simulink model "tailsitter2019b"  (R2019b)
settings: Solver=VariableStepAuto  StartTime=0.0  StopTime=10  RelTol=1e-3
values from neighbouring files (symbols this model uses):
  A_R = b^2/S    (= 3.125)    [tailsitterParam.m]
  b = [b1;b2;b3;b4;b5;b4;b3]    [tailsitterParam.m]
  c = [c1;c2;c3;c3;c3;c3;c3]    [tailsitterParam.m]
  C_D0 = 0.02    [tailsitterParam.m]
  C_D_R = 1.1    [tailsitterParam.m]
  C_M_coeff = polyfit(C_M_alpha(:,1), C_M_alpha(:,2),3)    [tailsitterParam.m]
  Cl_alpha = (2*pi*cos(Lambda))/(2*cos(Lambda)/A_R + sqrt(1 + (2*cos(Lambda)/A_R)^2))    [tailsitterParam.m]
  d = cat(2,p_d,p_d)    [tailsitterParam.m]
  g = -9.82    [tailsitterParam.m]
  Ic = [Ix 0 -Ixz;0 Iy 0;-Ixz 0 Iz]    [tailsitterParam.m]
  Initial_coeffs = polyfit(Thrusts_0,Omegas_0,4)    [tailsitterParam.m]
  Ith = 1.6*10^(-6)    (= 1.6e-06)    [tailsitterParam.m]
  k0 = 0.87    [tailsitterParam.m]
  l = 0.145    [tailsitterParam.m]
  li = cat(2,lr,ll)    [tailsitterParam.m]
  m = 0.21    [tailsitterParam.m]
  M_inv = inv(M)    [tailsitterParam.m]
  Omega_max = 1500    [tailsitterParam.m]
  pm = cat(2,prm,plm)    [tailsitterParam.m]
  r_B = r_B./1000    [tailsitterParam.m]
  R_eb = axang2rotm([0 1 0 -1.572])    [tailsitterParam.m]
  R_eleb1 = axang2rotm([0 0 1 -0.16349])    [tailsitterParam.m]
  R_eleb2 = axang2rotm([0 0 1 0.15331])    [tailsitterParam.m]
  rho = 1.225    [tailsitterParam.m]
  rp = 0.0625    [tailsitterParam.m]
  rv_B = rv_B./1000    [tailsitterParam.m]
  t_be = [0.5;0;0.5]    [tailsitterParam.m]
libraries: simulink x6, vrlib x1
settings Model: Creator=Thobi  LastModifiedBy=morten
settings DebuggingCC: SFMachineParentedDataDiag=error

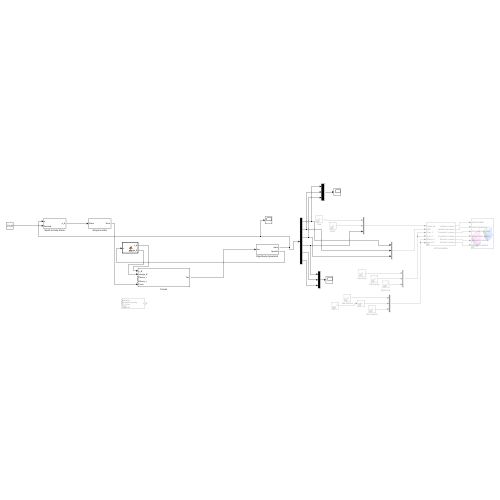
[thumbnail: Simulink's stored preview of the top-level diagram]
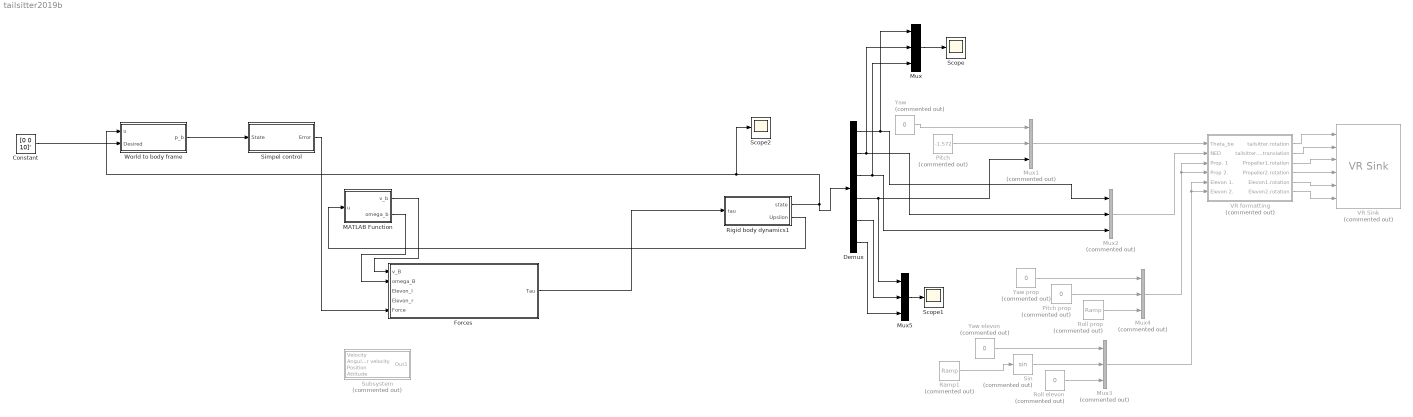
== system tailsitter2019b ==
  Constant : Constant  Value=[0 0 10]'
  Demux : Demux  Outputs=6
  Forces : Subsystem
  MATLAB Function : MATLAB Function  TreatAsAtomicUnit=on
  Mux : Mux  Inputs=3
  Mux{1..4} (4 alike) : Mux  Commented=on  Inputs=3
  Mux5 : Mux  Inputs=3
  Pitch : Constant  Commented=on  Value=-1.572
  Pitch prop : Constant  Commented=on  Value=0
  Ramp1 : simulink/Sources/Ramp  Commented=on  slope=1  start=0  InitialOutput=0
  Rigid body dynamics1 : Subsystem
  Roll elevon : Constant  Commented=on  Value=0
  Roll prop : simulink/Sources/Ramp  Commented=on  slope=1  start=0  InitialOutput=0
  Scope : Scope
  Scope1 : Scope
  Scope2 : Scope
  Simpel control : Subsystem
  Sin : Trigonometry  Commented=on
  Subsystem : Subsystem  Commented=on
  VR Sink : vrlib/VR Sink  Commented=on  InstantiateOnLoad=on  SampleTime=0.1  ViewEnable=on  RemoteChange=off  RemoteView=on  FieldsWritten=UAV.rotation.4.1.1.double#UAV.translation.3.1.1.double#Propeller1.rotation.4.1.1.double#Propeller2.rotation.4.1.1.double#Elevon1.rotation.4.1.1.double#Elevon2.rotation.4.1.1.double  WorldFileName=tailsitter_VR_simple.x3d  AutoView=off  VideoDimensions=[]  AllowVariableSize=off
  VR formatting : Subsystem  Commented=on
  World to body frame : Subsystem
  Yaw : Constant  Commented=on  Value=0
  Yaw elevon : Constant  Commented=on  Value=0
  Yaw prop : Constant  Commented=on  Value=0
  wires:
  VR formatting/5(Elevon1.rotation) -> VR Sink/5
  Roll prop/1 -> Mux4/3
  VR formatting/1(tailsitter.rotation) -> VR Sink/1
  Mux1/1 -> VR formatting/1(Theta_be)
  VR formatting/2(tailsitter.translation) -> VR Sink/2
  Sin/1 -> Mux3/2
  Roll elevon/1 -> Mux3/3
  Ramp1/1 -> Sin/1
  Yaw elevon/1 -> Mux3/1
  Mux3/1 -> VR formatting/6(Elevon 2.), VR formatting/5(Elevon 1.)
  Rigid body dynamics1/1(state) -> Demux/1, Scope2/1, World to body frame/1(u)
  Pitch/1 -> Mux1/2
  Demux/2 -> Mux/2, Mux2/2
  Mux2/1 -> VR formatting/2(NED)
  Yaw/1 -> Mux1/1
  VR formatting/6(Elevon2.rotation) -> VR Sink/6
  VR formatting/4(Propeller2.rotation) -> VR Sink/4
  Demux/4 -> Mux5/1, Mux1/3
  Yaw prop/1 -> Mux4/1
  Pitch prop/1 -> Mux4/2
  VR formatting/3(Propeller1.rotation) -> VR Sink/3
  Mux4/1 -> VR formatting/4(Prop 2.), VR formatting/3("Prop. 1 ")
  Simpel control/1(Error) -> Forces/5(Force)
  World to body frame/1(p_b) -> Simpel control/1(State)
  Rigid body dynamics1/2(Upsilon) -> MATLAB Function/1(u)
  MATLAB Function/1(v_b) -> Forces/1(v_B)
  MATLAB Function/2(omega_b) -> Forces/2(omega_B)
  Forces/1(Tau) -> Rigid body dynamics1/1(tau)
  Demux/1 -> Mux/1, Mux2/1
  Demux/3 -> Mux/3, Mux2/3
  Mux/1 -> Scope/1
  Demux/5 -> Mux5/2
  Demux/6 -> Mux5/3
  Mux5/1 -> Scope1/1
  Constant/1 -> World to body frame/2(Desired)

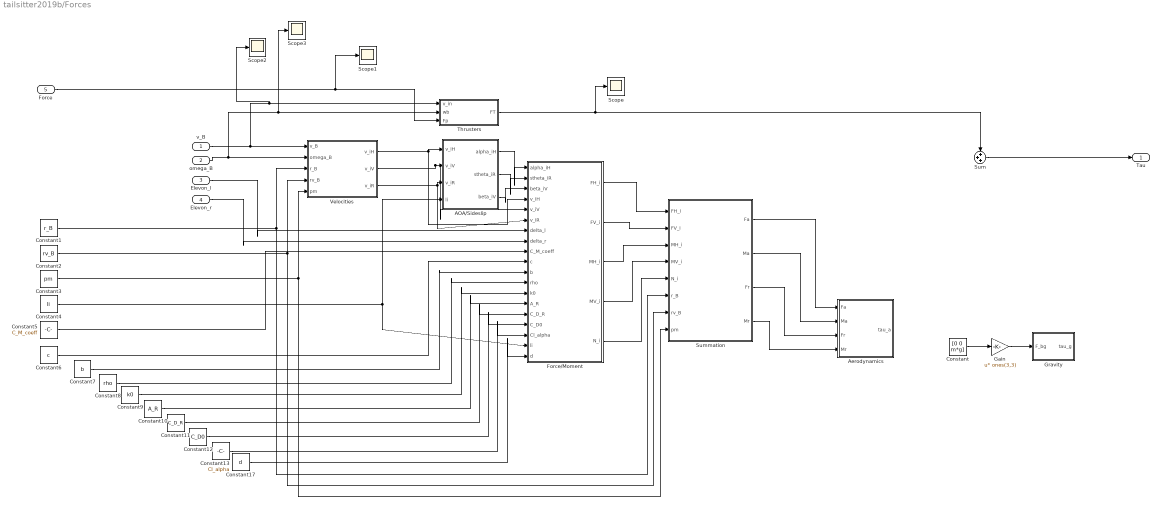
== system tailsitter2019b/Forces ==
  v_B : Inport
  omega_B : Inport  Port=2
  Elevon_l : Inport  Port=3
  Elevon_r : Inport  Port=4
  Force : Inport  Port=5
  AOA/Sideslip : MATLAB Function  TreatAsAtomicUnit=on
  Aerodynamics : MATLAB Function  TreatAsAtomicUnit=on
  Constant : Constant  Value=[0 0 m*g]
  Constant1 : Constant  Value=r_B
  Constant10 : Constant  Value=A_R
  Constant11 : Constant  Value=C_D_R
  Constant12 : Constant  Value=C_D0
  Constant13 : Constant  Value=Cl_alpha
  Constant17 : Constant  Value=d
  Constant2 : Constant  Value=rv_B
  Constant3 : Constant  Value=pm
  Constant4 : Constant  Value=li
  Constant5 : Constant  Value=C_M_coeff
  Constant6 : Constant  Value=c
  Constant7 : Constant  Value=b
  Constant8 : Constant  Value=rho
  Constant9 : Constant  Value=k0
  Force/Moment : MATLAB Function  TreatAsAtomicUnit=on
  Gain : Gain  Gain=ones(3,3)  Multiplication=Matrix(u*K)
  Gravity : MATLAB Function  TreatAsAtomicUnit=on
  Scope{,1..3} (4 alike) : Scope
  Sum : Sum  Inputs=+++
  Summation : MATLAB Function  TreatAsAtomicUnit=on
  Thrusters : Subsystem
  Velocities : MATLAB Function  TreatAsAtomicUnit=on
  Tau : Outport
  wires:
  v_B/1 -> Scope2/1, Thrusters/1(v_in), Velocities/1(v_B)
  Gain/1 -> Gravity/1(F_bg)
  Velocities/1(v_iH) -> AOA/Sideslip/1(v_iH), Force/Moment/4(v_iH)
  Velocities/2(v_iV) -> Force/Moment/5(v_iV), AOA/Sideslip/2(v_iV)
  Velocities/3(v_iR) -> Force/Moment/6(v_iR), AOA/Sideslip/3(v_iR)
  AOA/Sideslip/1(alpha_iH) -> Force/Moment/1(alpha_iH)
  AOA/Sideslip/2(stheta_iR) -> Force/Moment/2(stheta_iR)
  AOA/Sideslip/3(beta_iV) -> Force/Moment/3(beta_iV)
  Force/Moment/1(FH_i) -> Summation/1(FH_i)
  Force/Moment/2(FV_i) -> Summation/2(FV_i)
  Force/Moment/3(MH_i) -> Summation/3(MH_i)
  Force/Moment/4(MV_i) -> Summation/4(MV_i)
  Force/Moment/5(N_i) -> Summation/5(N_i)
  Summation/1(Fa) -> Aerodynamics/1(Fa)
  Summation/2(Ma) -> Aerodynamics/2(Ma)
  Summation/3(Fr) -> Aerodynamics/3(Fr)
  Summation/4(Mr) -> Aerodynamics/4(Mr)
  Sum/1 -> Tau/1
  Elevon_l/1 -> Force/Moment/7(delta_l)
  Elevon_r/1 -> Force/Moment/8(delta_r)
  Constant/1 -> Gain/1
  Constant1/1 -> Summation/6(r_B), Velocities/3(r_B)
  Constant2/1 -> Velocities/4(rv_B), Summation/7(rv_B)
  Constant3/1 -> Velocities/5(pm), Summation/8(pm)
  Constant4/1 -> Force/Moment/18(li), AOA/Sideslip/4(li)
  Constant5/1 -> Force/Moment/9(C_M_coeff)
  Constant6/1 -> Force/Moment/10(c)
  Constant7/1 -> Force/Moment/11(b)
  Constant8/1 -> Force/Moment/12(rho)
  Constant9/1 -> Force/Moment/13(k0)
  Constant10/1 -> Force/Moment/14(A_R)
  Constant11/1 -> Force/Moment/15(C_D_R)
  Constant12/1 -> Force/Moment/16(C_D0)
  Constant13/1 -> Force/Moment/17(Cl_alpha)
  Thrusters/1(FT) -> Scope/1, Sum/1
  Constant17/1 -> Force/Moment/19(d)
  Force/1 -> Scope1/1, Thrusters/3(Fp)
  omega_B/1 -> Thrusters/2(wb), Scope3/1, Velocities/2(omega_B)

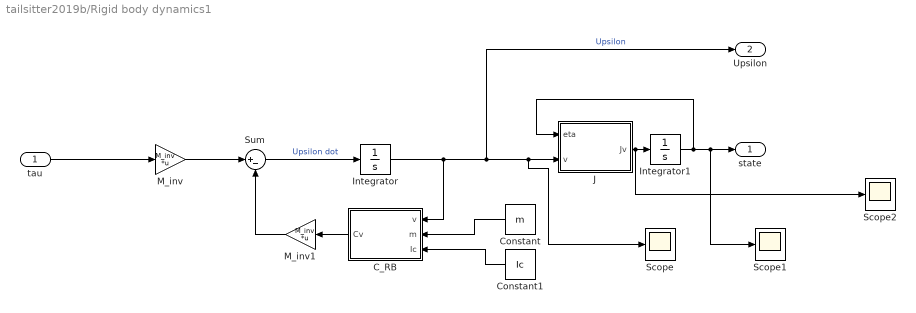
== system tailsitter2019b/Rigid body dynamics1 ==
  tau : Inport
  C_RB : MATLAB Function  TreatAsAtomicUnit=on
  Constant : Constant  Value=m
  Constant1 : Constant  Value=Ic
  Integrator : Integrator  InitialCondition=[0;0;0;0;0;0]
  Integrator1 : Integrator  InitialCondition=[0;0;0;0;-pi/2;0]
  J : MATLAB Function  TreatAsAtomicUnit=on
  M_inv : Gain  Gain=M_inv  Multiplication=Matrix(K*u) (u vector)
  M_inv1 : Gain  Gain=M_inv  Multiplication=Matrix(K*u) (u vector)
  Scope : Scope
  Scope1 : Scope
  Scope2 : Scope
  Sum : Sum  Inputs=|+-
  state : Outport
  Upsilon : Outport  Port=2
  wires:
  tau/1 -> M_inv/1
  M_inv/1 -> Sum/1
  Sum/1 -> Integrator/1  "Upsilon dot"
  C_RB/1(Cv) -> M_inv1/1
  M_inv1/1 -> Sum/2
  Integrator/1 -> C_RB/1(v), Upsilon/1, Scope/1, J/2(v)  "Upsilon"
  Constant/1 -> C_RB/2(m)
  Constant1/1 -> C_RB/3(Ic)
  J/1(Jv) -> Scope2/1, Integrator1/1
  Integrator1/1 -> Scope1/1, state/1, J/1(eta)

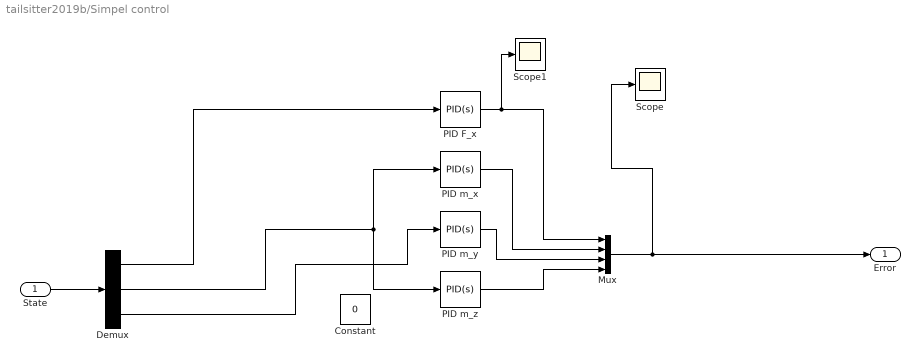
== system tailsitter2019b/Simpel control ==
  State : Inport
  Constant : Constant  Value=0
  Demux : Demux  Outputs=3
  Mux : Mux
  PID F_x : simulink/Continuous/PID Controller  Controller=PID  Form=Parallel  TimeDomain=Continuous-time  SampleTime=-1  IntegratorMethod=Forward Euler  ControllerParametersSource=internal  P=1.2  I=1  D=0  UseFilter=on  N=100  TunerSelectOption=Transfer Function Based (PID Tuner App)  InitialConditionSource=internal  InitialConditionForIntegrator=0  InitialConditionForFilter=0  DifferentiatorICPrevScaledInput=0  ExternalReset=none  TrackingMode=off  Kt=1  LimitOutput=off  UpperSaturationLimit=inf  LowerSaturationLimit=-inf  LinearizeAsGain=on  AntiWindupMode=none  Kb=1  POutMin=[]  POutMax=[]  IOutMin=[]  IOutMax=[]  DOutMin=[]  DOutMax=[]  NOutMin=[]  NOutMax=[]  SumOutMin=[]  SumOutMax=[]  SaturationOutMin=[]  SaturationOutMax=[]  PParamMin=[]  PParamMax=[]  IParamMin=[]  IParamMax=[]  DParamMin=[]  DParamMax=[]  NParamMin=[]  NParamMax=[]  KbParamMin=[]  KbParamMax=[]  KtParamMin=[]  KtParamMax=[]  KbOutMin=[]  KbOutMax=[]  KtOutMin=[]  KtOutMax=[]  IntegratorOutMin=[]  IntegratorOutMax=[]  FilterOutMin=[]  FilterOutMax=[]  SumI1OutMin=[]  SumI1OutMax=[]  SumI2OutMin=[]  SumI2OutMax=[]  SumI3OutMin=[]  SumI3OutMax=[]  SumI4OutMin=[]  SumI4OutMax=[]  SumDOutMin=[]  SumDOutMax=[]  DifferentiatorOutMin=[]  DifferentiatorOutMax=[]  FilterDiffOutCoefMin=[]  FilterDiffOutCoefMax=[]  ReciprocalOutMin=[]  ReciprocalOutMax=[]  SumDenOutMin=[]  SumDenOutMax=[]  SumNumOutMin=[]  SumNumOutMax=[]  DivideOutMin=[]  DivideOutMax=[]  IntegratorContinuousStateAttributes=''  IntegratorStateMustResolveToSignalObject=off  IntegratorRTWStateStorageClass=Auto  FilterContinuousStateAttributes=''  FilterStateMustResolveToSignalObject=off  FilterRTWStateStorageClass=Auto  ParallelPVariant=InternalParameters  IdealPVariant=Disabled  IVariant=InternalParameters  DVariant=InternalParameters  IntegratorVariant=Continuous  SatVariant=Disabled  AWVariant=Passthrough  PCopyVariant=Disabled  TRVariant=Disabled  FdbkBlocksVariant=Forward  IdealPFdbkVariant=Disabled  SatFdbkVariant=Disabled  DerivativeFilterVariant=ContFilter  NVariant=InternalParameters  NCopyVariant=Disabled  FilterICVariant=InternalICsFilter  IntegratorICVariant=InternalICs  ExternalResetVariant=Disabled  TRSumVariant=Passthrough  SumFdbkVariant=Disabled  SumVariant=Sum_PID
  PID m_x : simulink/Continuous/PID Controller  Controller=PID  Form=Parallel  TimeDomain=Continuous-time  SampleTime=-1  IntegratorMethod=Forward Euler  ControllerParametersSource=internal  P=1.2  I=1  D=0  UseFilter=on  N=100  TunerSelectOption=Transfer Function Based (PID Tuner App)  InitialConditionSource=internal  InitialConditionForIntegrator=0  InitialConditionForFilter=0  DifferentiatorICPrevScaledInput=0  ExternalReset=none  TrackingMode=off  Kt=1  LimitOutput=off  UpperSaturationLimit=inf  LowerSaturationLimit=-inf  LinearizeAsGain=on  AntiWindupMode=none  Kb=1  POutMin=[]  POutMax=[]  IOutMin=[]  IOutMax=[]  DOutMin=[]  DOutMax=[]  NOutMin=[]  NOutMax=[]  SumOutMin=[]  SumOutMax=[]  SaturationOutMin=[]  SaturationOutMax=[]  PParamMin=[]  PParamMax=[]  IParamMin=[]  IParamMax=[]  DParamMin=[]  DParamMax=[]  NParamMin=[]  NParamMax=[]  KbParamMin=[]  KbParamMax=[]  KtParamMin=[]  KtParamMax=[]  KbOutMin=[]  KbOutMax=[]  KtOutMin=[]  KtOutMax=[]  IntegratorOutMin=[]  IntegratorOutMax=[]  FilterOutMin=[]  FilterOutMax=[]  SumI1OutMin=[]  SumI1OutMax=[]  SumI2OutMin=[]  SumI2OutMax=[]  SumI3OutMin=[]  SumI3OutMax=[]  SumI4OutMin=[]  SumI4OutMax=[]  SumDOutMin=[]  SumDOutMax=[]  DifferentiatorOutMin=[]  DifferentiatorOutMax=[]  FilterDiffOutCoefMin=[]  FilterDiffOutCoefMax=[]  ReciprocalOutMin=[]  ReciprocalOutMax=[]  SumDenOutMin=[]  SumDenOutMax=[]  SumNumOutMin=[]  SumNumOutMax=[]  DivideOutMin=[]  DivideOutMax=[]  IntegratorContinuousStateAttributes=''  IntegratorStateMustResolveToSignalObject=off  IntegratorRTWStateStorageClass=Auto  FilterContinuousStateAttributes=''  FilterStateMustResolveToSignalObject=off  FilterRTWStateStorageClass=Auto  ParallelPVariant=InternalParameters  IdealPVariant=Disabled  IVariant=InternalParameters  DVariant=InternalParameters  IntegratorVariant=Continuous  SatVariant=Disabled  AWVariant=Passthrough  PCopyVariant=Disabled  TRVariant=Disabled  FdbkBlocksVariant=Forward  IdealPFdbkVariant=Disabled  SatFdbkVariant=Disabled  DerivativeFilterVariant=ContFilter  NVariant=InternalParameters  NCopyVariant=Disabled  FilterICVariant=InternalICsFilter  IntegratorICVariant=InternalICs  ExternalResetVariant=Disabled  TRSumVariant=Passthrough  SumFdbkVariant=Disabled  SumVariant=Sum_PID
  PID m_y : simulink/Continuous/PID Controller  Controller=PID  Form=Parallel  TimeDomain=Continuous-time  SampleTime=-1  IntegratorMethod=Forward Euler  ControllerParametersSource=internal  P=1.2  I=1  D=0  UseFilter=on  N=100  TunerSelectOption=Transfer Function Based (PID Tuner App)  InitialConditionSource=internal  InitialConditionForIntegrator=0  InitialConditionForFilter=0  DifferentiatorICPrevScaledInput=0  ExternalReset=none  TrackingMode=off  Kt=1  LimitOutput=off  UpperSaturationLimit=inf  LowerSaturationLimit=-inf  LinearizeAsGain=on  AntiWindupMode=none  Kb=1  POutMin=[]  POutMax=[]  IOutMin=[]  IOutMax=[]  DOutMin=[]  DOutMax=[]  NOutMin=[]  NOutMax=[]  SumOutMin=[]  SumOutMax=[]  SaturationOutMin=[]  SaturationOutMax=[]  PParamMin=[]  PParamMax=[]  IParamMin=[]  IParamMax=[]  DParamMin=[]  DParamMax=[]  NParamMin=[]  NParamMax=[]  KbParamMin=[]  KbParamMax=[]  KtParamMin=[]  KtParamMax=[]  KbOutMin=[]  KbOutMax=[]  KtOutMin=[]  KtOutMax=[]  IntegratorOutMin=[]  IntegratorOutMax=[]  FilterOutMin=[]  FilterOutMax=[]  SumI1OutMin=[]  SumI1OutMax=[]  SumI2OutMin=[]  SumI2OutMax=[]  SumI3OutMin=[]  SumI3OutMax=[]  SumI4OutMin=[]  SumI4OutMax=[]  SumDOutMin=[]  SumDOutMax=[]  DifferentiatorOutMin=[]  DifferentiatorOutMax=[]  FilterDiffOutCoefMin=[]  FilterDiffOutCoefMax=[]  ReciprocalOutMin=[]  ReciprocalOutMax=[]  SumDenOutMin=[]  SumDenOutMax=[]  SumNumOutMin=[]  SumNumOutMax=[]  DivideOutMin=[]  DivideOutMax=[]  IntegratorContinuousStateAttributes=''  IntegratorStateMustResolveToSignalObject=off  IntegratorRTWStateStorageClass=Auto  FilterContinuousStateAttributes=''  FilterStateMustResolveToSignalObject=off  FilterRTWStateStorageClass=Auto  ParallelPVariant=InternalParameters  IdealPVariant=Disabled  IVariant=InternalParameters  DVariant=InternalParameters  IntegratorVariant=Continuous  SatVariant=Disabled  AWVariant=Passthrough  PCopyVariant=Disabled  TRVariant=Disabled  FdbkBlocksVariant=Forward  IdealPFdbkVariant=Disabled  SatFdbkVariant=Disabled  DerivativeFilterVariant=ContFilter  NVariant=InternalParameters  NCopyVariant=Disabled  FilterICVariant=InternalICsFilter  IntegratorICVariant=InternalICs  ExternalResetVariant=Disabled  TRSumVariant=Passthrough  SumFdbkVariant=Disabled  SumVariant=Sum_PID
  PID m_z : simulink/Continuous/PID Controller  Controller=PID  Form=Parallel  TimeDomain=Continuous-time  SampleTime=-1  IntegratorMethod=Forward Euler  ControllerParametersSource=internal  P=1.2  I=1  D=0  UseFilter=on  N=100  TunerSelectOption=Transfer Function Based (PID Tuner App)  InitialConditionSource=internal  InitialConditionForIntegrator=0  InitialConditionForFilter=0  DifferentiatorICPrevScaledInput=0  ExternalReset=none  TrackingMode=off  Kt=1  LimitOutput=off  UpperSaturationLimit=inf  LowerSaturationLimit=-inf  LinearizeAsGain=on  AntiWindupMode=none  Kb=1  POutMin=[]  POutMax=[]  IOutMin=[]  IOutMax=[]  DOutMin=[]  DOutMax=[]  NOutMin=[]  NOutMax=[]  SumOutMin=[]  SumOutMax=[]  SaturationOutMin=[]  SaturationOutMax=[]  PParamMin=[]  PParamMax=[]  IParamMin=[]  IParamMax=[]  DParamMin=[]  DParamMax=[]  NParamMin=[]  NParamMax=[]  KbParamMin=[]  KbParamMax=[]  KtParamMin=[]  KtParamMax=[]  KbOutMin=[]  KbOutMax=[]  KtOutMin=[]  KtOutMax=[]  IntegratorOutMin=[]  IntegratorOutMax=[]  FilterOutMin=[]  FilterOutMax=[]  SumI1OutMin=[]  SumI1OutMax=[]  SumI2OutMin=[]  SumI2OutMax=[]  SumI3OutMin=[]  SumI3OutMax=[]  SumI4OutMin=[]  SumI4OutMax=[]  SumDOutMin=[]  SumDOutMax=[]  DifferentiatorOutMin=[]  DifferentiatorOutMax=[]  FilterDiffOutCoefMin=[]  FilterDiffOutCoefMax=[]  ReciprocalOutMin=[]  ReciprocalOutMax=[]  SumDenOutMin=[]  SumDenOutMax=[]  SumNumOutMin=[]  SumNumOutMax=[]  DivideOutMin=[]  DivideOutMax=[]  IntegratorContinuousStateAttributes=''  IntegratorStateMustResolveToSignalObject=off  IntegratorRTWStateStorageClass=Auto  FilterContinuousStateAttributes=''  FilterStateMustResolveToSignalObject=off  FilterRTWStateStorageClass=Auto  ParallelPVariant=InternalParameters  IdealPVariant=Disabled  IVariant=InternalParameters  DVariant=InternalParameters  IntegratorVariant=Continuous  SatVariant=Disabled  AWVariant=Passthrough  PCopyVariant=Disabled  TRVariant=Disabled  FdbkBlocksVariant=Forward  IdealPFdbkVariant=Disabled  SatFdbkVariant=Disabled  DerivativeFilterVariant=ContFilter  NVariant=InternalParameters  NCopyVariant=Disabled  FilterICVariant=InternalICsFilter  IntegratorICVariant=InternalICs  ExternalResetVariant=Disabled  TRSumVariant=Passthrough  SumFdbkVariant=Disabled  SumVariant=Sum_PID
  Scope : Scope
  Scope1 : Scope
  Error : Outport
  wires:
  Mux/1 -> Scope/1, Error/1
  Demux/1 -> PID F_x/1
  State/1 -> Demux/1
  Demux/2 -> PID m_z/1, PID m_x/1
  Demux/3 -> PID m_y/1
  PID F_x/1 -> Scope1/1, Mux/1
  PID m_x/1 -> Mux/2
  PID m_y/1 -> Mux/3
  PID m_z/1 -> Mux/4

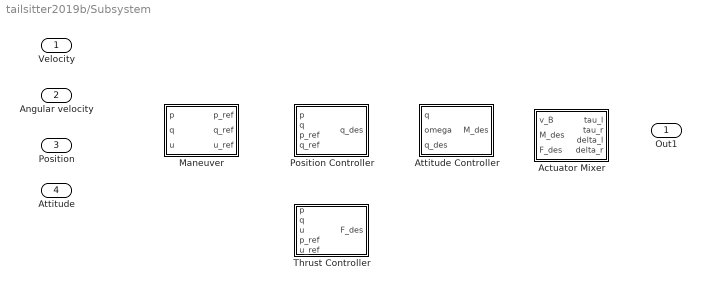
== system tailsitter2019b/Subsystem ==
  Velocity : Inport
  Angular velocity : Inport  Port=2
  Position : Inport  Port=3
  Attitude : Inport  Port=4
  Actuator Mixer : MATLAB Function  TreatAsAtomicUnit=on
  Attitude Controller : MATLAB Function  TreatAsAtomicUnit=on
  Maneuver : MATLAB Function  TreatAsAtomicUnit=on
  Position Controller : MATLAB Function  TreatAsAtomicUnit=on
  Thrust Controller : MATLAB Function  TreatAsAtomicUnit=on
  Out1 : Outport

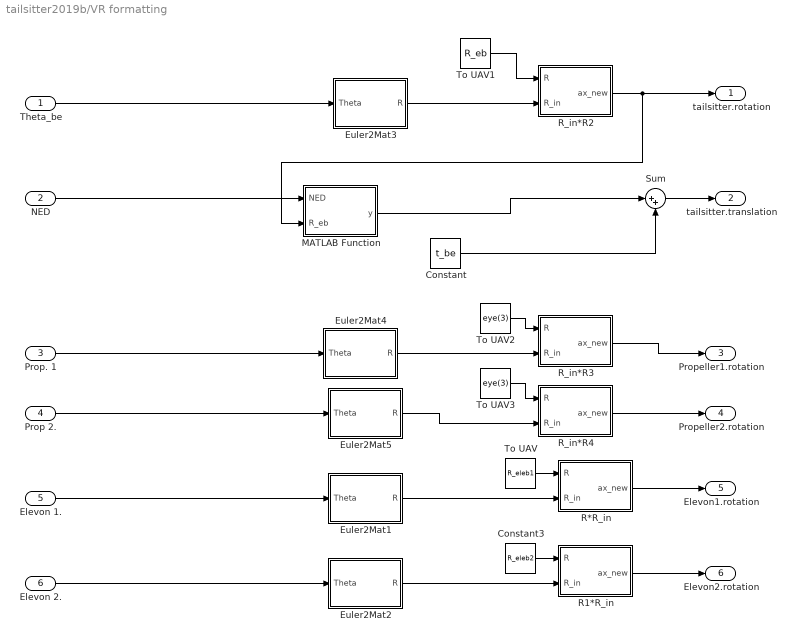
== system tailsitter2019b/VR formatting ==
  Theta_be : Inport
  NED : Inport  Port=2
  "Prop. 1 " : Inport  Port=3
  Prop 2. : Inport  Port=4
  Elevon 1. : Inport  Port=5
  Elevon 2. : Inport  Port=6
  Constant : Constant  Value=t_be
  Constant3 : Constant  Value=R_eleb2
  Euler2Mat1 : MATLAB Function  TreatAsAtomicUnit=on
  Euler2Mat2 : MATLAB Function  TreatAsAtomicUnit=on
  Euler2Mat3 : MATLAB Function  TreatAsAtomicUnit=on
  Euler2Mat4 : MATLAB Function  TreatAsAtomicUnit=on
  Euler2Mat5 : MATLAB Function  TreatAsAtomicUnit=on
  MATLAB Function : MATLAB Function  TreatAsAtomicUnit=on
  R*R_in : MATLAB Function  TreatAsAtomicUnit=on
  R1*R_in : MATLAB Function  TreatAsAtomicUnit=on
  R_in*R2 : MATLAB Function  TreatAsAtomicUnit=on
  R_in*R3 : MATLAB Function  TreatAsAtomicUnit=on
  R_in*R4 : MATLAB Function  TreatAsAtomicUnit=on
  Sum : Sum  Inputs=|++
  To UAV : Constant  Value=R_eleb1
  To UAV1 : Constant  Value=R_eb
  To UAV2 : Constant  Value=eye(3)
  To UAV3 : Constant  Value=eye(3)
  tailsitter.rotation : Outport
  tailsitter.translation : Outport  Port=2
  Propeller1.rotation : Outport  Port=3
  Propeller2.rotation : Outport  Port=4
  Elevon1.rotation : Outport  Port=5
  Elevon2.rotation : Outport  Port=6
  wires:
  NED/1 -> MATLAB Function/1(NED)
  Theta_be/1 -> Euler2Mat3/1(Theta)
  MATLAB Function/1(y) -> Sum/1
  Sum/1 -> tailsitter.translation/1
  Constant/1 -> Sum/2
  "Prop. 1 "/1 -> Euler2Mat4/1(Theta)
  Elevon 1./1 -> Euler2Mat1/1(Theta)
  Elevon 2./1 -> Euler2Mat2/1(Theta)
  Euler2Mat1/1(R) -> R*R_in/2(R_in)
  To UAV/1 -> R*R_in/1(R)
  R*R_in/1(ax_new) -> Elevon1.rotation/1
  Euler2Mat2/1(R) -> R1*R_in/2(R_in)
  R1*R_in/1(ax_new) -> Elevon2.rotation/1
  Constant3/1 -> R1*R_in/1(R)
  Euler2Mat3/1(R) -> R_in*R2/2(R_in)
  R_in*R2/1(ax_new) -> MATLAB Function/2(R_eb), tailsitter.rotation/1
  To UAV1/1 -> R_in*R2/1(R)
  To UAV2/1 -> R_in*R3/1(R)
  Euler2Mat4/1(R) -> R_in*R3/2(R_in)
  R_in*R3/1(ax_new) -> Propeller1.rotation/1
  Prop 2./1 -> Euler2Mat5/1(Theta)
  R_in*R4/1(ax_new) -> Propeller2.rotation/1
  To UAV3/1 -> R_in*R4/1(R)
  Euler2Mat5/1(R) -> R_in*R4/2(R_in)

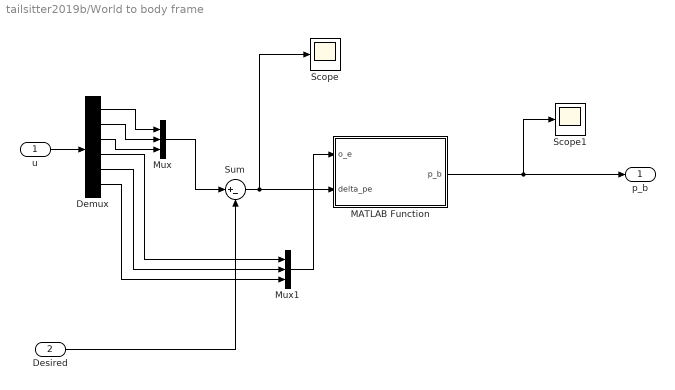
== system tailsitter2019b/World to body frame ==
  u : Inport
  Desired : Inport  Port=2
  Demux : Demux  Outputs=6
  MATLAB Function : MATLAB Function  TreatAsAtomicUnit=on
  Mux : Mux  Inputs=3
  Mux1 : Mux  Inputs=3
  Scope : Scope
  Scope1 : Scope
  Sum : Sum  Inputs=|+-
  p_b : Outport
  wires:
  MATLAB Function/1(p_b) -> Scope1/1, p_b/1
  Desired/1 -> Sum/2
  u/1 -> Demux/1
  Mux/1 -> Sum/1
  Demux/1 -> Mux/1
  Demux/2 -> Mux/2
  Demux/3 -> Mux/3
  Demux/4 -> Mux1/1
  Demux/5 -> Mux1/2
  Demux/6 -> Mux1/3
  Mux1/1 -> MATLAB Function/1(o_e)
  Sum/1 -> Scope/1, MATLAB Function/2(delta_pe)

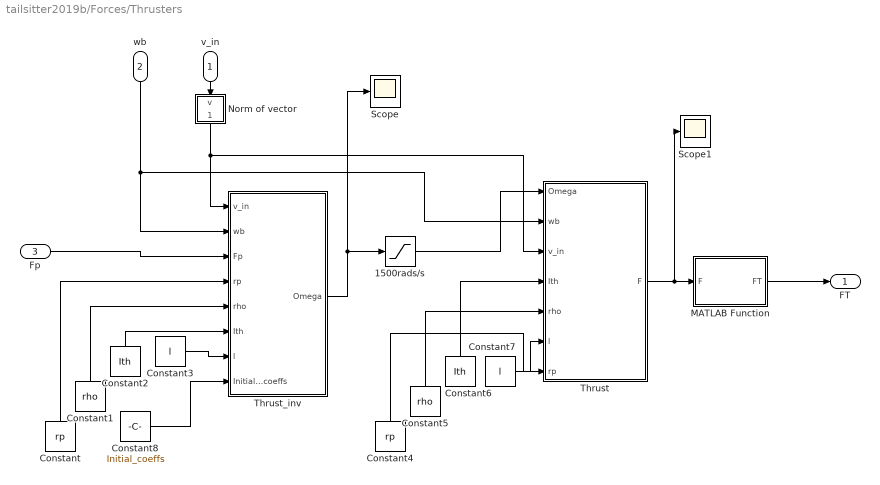
== system tailsitter2019b/Forces/Thrusters ==
  v_in : Inport
  wb : Inport  Port=2
  Fp : Inport  Port=3  PortDimensions=4
  1500rads/s : Saturate  UpperLimit=Omega_max  LowerLimit=-Omega_max
  Constant : Constant  Value=rp
  Constant1 : Constant  Value=rho
  Constant2 : Constant  Value=Ith
  Constant3 : Constant  Value=l
  Constant4 : Constant  Value=rp
  Constant5 : Constant  Value=rho
  Constant6 : Constant  Value=Ith
  Constant7 : Constant  Value=l
  Constant8 : Constant  Value=Initial_coeffs
  MATLAB Function : MATLAB Function  TreatAsAtomicUnit=on
  Norm of vector : MATLAB Function  TreatAsAtomicUnit=on
  Scope : Scope
  Scope1 : Scope
  Thrust : MATLAB Function  TreatAsAtomicUnit=on
  Thrust_inv : MATLAB Function  TreatAsAtomicUnit=on
  FT : Outport
  wires:
  Thrust/1(F) -> Scope1/1, MATLAB Function/1(F)
  Fp/1 -> Thrust_inv/3(Fp)
  Thrust_inv/1(Omega) -> Scope/1, 1500rads/s/1
  wb/1 -> Thrust/2(wb), Thrust_inv/2(wb)
  Constant/1 -> Thrust_inv/4(rp)
  Constant1/1 -> Thrust_inv/5(rho)
  Constant2/1 -> Thrust_inv/6(Ith)
  Constant3/1 -> Thrust_inv/7(l)
  Constant4/1 -> Thrust/7(rp)
  Constant5/1 -> Thrust/5(rho)
  Constant6/1 -> Thrust/4(Ith)
  Constant7/1 -> Thrust/6(l)
  MATLAB Function/1(FT) -> FT/1
  v_in/1 -> Norm of vector/1(v)
  Norm of vector/1(v_norm) -> Thrust/3(v_in), Thrust_inv/1(v_in)
  1500rads/s/1 -> Thrust/1(Omega)
  Constant8/1 -> Thrust_inv/8(Initial_coeffs)

== matlab function tailsitter2019b/MATLAB Function ==
  data: u input; v_b output; omega_b output
function [v_b, omega_b] = fcn(u)

    v_b = zeros(3,1);
    v_b = u(1:3);

    omega_b = u(4:6);

end

== matlab function tailsitter2019b/World to body frame/MATLAB Function ==
  data: o_e input; p_b output; delta_pe input
function p_b = fcn(o_e, delta_pe)

    p_b = zeros(3,1);


    p_b = eul2rotm([o_e(3) o_e(2) o_e(1)])'*delta_pe;

end

== matlab function tailsitter2019b/Rigid body dynamics1/C_RB ==
  data: v input; m input; Ic input; Cv output
function Cv = fcn(v, m, Ic)
    w = v(4:6,1);
    w_cross = [0 -w(3) w(2);w(3) 0 -w(1);-w(2) w(1) 0];
    Ic_w = Ic*w;    
    Ic_w_cross = [0 -Ic_w(3) Ic_w(2);Ic_w(3) 0 -Ic_w(1);-Ic_w(2) Ic_w(1) 0];
    C = [m*w_cross zeros(3,3);zeros(3,3) -Ic_w_cross];
    Cv = C*v;
end

== matlab function tailsitter2019b/Rigid body dynamics1/J ==
  data: eta input; Jv output; v input
function Jv = fcn(eta, v)
    %R = eul2rotm(eta(4:6), "ZYX");

    phi = eta(4);
    theta = eta(5);
    psi = eta(6);
    Rx = [1 0 0; 0 cos(phi) -sin(phi); 0 sin(phi) cos(phi)];
    Ry = [cos(theta) 0 sin(theta); 0 1 0; -sin(theta) 0 cos(theta)];
    Rz = [cos(psi) -sin(psi) 0; sin(psi) cos(psi) 0; 0 0 1];

    R = Rz*Ry*Rx;
    T = [1 sin(phi)*sin(theta)/cos(theta) cos(phi)*sin(theta)/cos(theta);0 cos(phi) -sin(phi);0 sin(phi)/cos(theta) cos(phi)/cos(theta)];
    J = [R zeros(3);zeros(3) T];

    Jv = J * v;

end

== matlab function tailsitter2019b/VR formatting/Euler2Mat1 ==
  data: Theta input; R output
function R = fcn(Theta)
R = eul2rotm(Theta', "ZYX"); %YAW - PITCH - ROLL
end

== matlab function tailsitter2019b/VR formatting/Euler2Mat3 ==
  data: Theta input; R output
function R = fcn(Theta)
R = eul2rotm(Theta', "ZYX"); %YAW - PITCH - ROLL
end

== matlab function tailsitter2019b/VR formatting/Euler2Mat2 ==
  data: Theta input; R output
function R = fcn(Theta)
R = eul2rotm(Theta', "ZYX"); %YAW - PITCH - ROLL
end

== matlab function tailsitter2019b/VR formatting/Euler2Mat4 ==
  data: Theta input; R output
function R = fcn(Theta)
R = eul2rotm(Theta', "ZYX"); %YAW - PITCH - ROLL
end

== matlab function tailsitter2019b/Subsystem/Maneuver ==
  data: p input; q input; u input; p_ref output; q_ref output; u_ref output
function [p_ref, q_ref, u_ref] = fcn(p, q, u)

end

== matlab function tailsitter2019b/Subsystem/Position Controller ==
  data: p input; q_des output; q input; p_ref input; q_ref input
function q_des = fcn(p, q, p_ref, q_ref)

end

== matlab function tailsitter2019b/Subsystem/Attitude Controller ==
  data: q input; M_des output; omega input; q_des input
function M_des = fcn(q, omega, q_des)

end

== matlab function tailsitter2019b/Forces/Gravity ==
  data: F_bg input; tau_g output
function tau_g = fcn(F_bg)

    tau_g = zeros(6,1);
    tau_g(1:3,1) = F_bg;
    

end

== matlab function tailsitter2019b/Subsystem/Thrust Controller ==
  data: p input; q input; u input; F_des output; p_ref input; u_ref input
function F_des = fcn(p, q, u, p_ref, u_ref)

end

== matlab function tailsitter2019b/Subsystem/Actuator Mixer ==
  data: v_B input; tau_l output; M_des input; F_des input; tau_r output; delta_l output; delta_r output
function [tau_l, tau_r, delta_l, delta_r] = fcn(v_B, M_des, F_des)

end

== matlab function tailsitter2019b/Forces/Velocities ==
  data: v_B input; v_iH output; omega_B input; v_iV output; v_iR output; r_B input; rv_B input; pm input
function [v_iH, v_iV, v_iR] = fcn(v_B,omega_B, r_B, rv_B, pm)
    v_w = 0;
    v_iH = zeros(3, size(r_B,2));
    for i = 1:size(r_B,2)
        v_iH(:,i) = v_B + cross(omega_B,r_B(:,i)) + v_w;
    end
    
    v_iV = zeros(3, size(rv_B,2));
    for i = 1:size(rv_B,2)
        v_iV(:,i) = v_B + cross(omega_B,rv_B(:,i)) + v_w;
    end
    
    v_iR = zeros(3, size(pm,2));
    for i = 1:size(pm,2)
        v_iR(:,i) = v_B + cross(omega_B,pm(:,i)) + v_w;
    end
    

end

== matlab function tailsitter2019b/Forces/AOA//Sideslip ==
  data: v_iH input; alpha_iH output; v_iV input; v_iR input; stheta_iR output; beta_iV output; li input
function [alpha_iH, stheta_iR, beta_iV] = fcn(v_iH, v_iV, v_iR, li)

    alpha_iH = zeros(size(v_iH,2),1);
    for i = 1:size(v_iH,2)
        alpha_iH(i) = atan2(v_iH(3,i),v_iH(1,i));
    end
    
    beta_iV = zeros(size(v_iV,2),1);
    for i = 1:size(v_iV,2)
        beta_iV(i) = atan2(v_iV(2,i),v_iV(1,i));
    end
    
    stheta_iR = zeros(size(v_iR,2),1);
    if norm(v_iR) == 0
        stheta_iR = zeros(size(v_iR,2),1);
    else
        for i = 1:size(v_iR,2)
            stheta_iR(i) = (norm(cross(v_iR(:,i),li(:,i))))/(norm(v_iR(:,i))*norm(li(:,i)));
        end
    end
end

== matlab function tailsitter2019b/Forces/Force//Moment ==
  data: alpha_iH input; stheta_iR input; beta_iV input; FH_i output; v_iH input; v_iV input; FV_i output; MH_i output; MV_i output; N_i output; v_iR input; delta_l input; delta_r input; C_M_coeff input; c input; b input; rho input; k0 input; A_R input; C_D_R input; C_D0 input; Cl_alpha input; li input; d input
function [FH_i, FV_i, MH_i, MV_i, N_i] = fcn(alpha_iH, stheta_iR, beta_iV, v_iH, v_iV, v_iR, delta_l, delta_r, C_M_coeff, c, b, rho, k0, A_R, C_D_R, C_D0, Cl_alpha, li, d)
    CL = 0;
    FH_i = zeros(3,size(alpha_iH,1));
    MH_i = zeros(3,size(alpha_iH,1));
    for i = 1:size(alpha_iH,1)
        if i == 4
            CL = Cl_alpha*(alpha_iH(1)+delta_l);
        elseif i == 6
            CL = Cl_alpha*(alpha_iH(1)+delta_r);
        else
            CL = Cl_alpha*alpha_iH(1);
        end
        CD = C_D0 + (CL^2)/(pi*k0*A_R);
        FHba_i = [CL*sin(alpha_iH(i))-CD*cos(alpha_iH(i)); 0; -CL*cos(alpha_iH(i))-CD*sin(alpha_iH(i))];
        FH_i(:,i) = (1/2)*rho*b(i)*c(i)*(v_iH(1,i)^2+v_iH(3,i)^2)*FHba_i;
        
        MH_i(:,i) = (1/2)*rho*b(i)*c(i)^2*(v_iH(1,i)^2+v_iH(3,i)^2)*(sum(C_M_coeff*alpha_iH(i)));
    end
    
    CL = 0;
    FV_i = zeros(3,size(beta_iV,1));
    MV_i = zeros(3,size(beta_iV,1));
    for i = 1:size(beta_iV,1)
        CL = Cl_alpha*alpha_iH(1);
        CD = C_D0 + (CL^2)/(pi*k0*A_R);
        FVba_i = [CL*sin(beta_iV(i))-CD*cos(beta_iV(i)); -CL*cos(beta_iV(i))-CD*sin(beta_iV(i)); 0];
        FV_i(:,i) = (1/2)*rho*b(i)*c(i)*(v_iV(1,i)^2+v_iV(2,i))*FVba_i;
        
        MV_i(:,i) = (1/2)*rho*b(i)*c(i)^2*(v_iV(1,i)^2+v_iV(2,i)^2)*(sum(C_M_coeff*alpha_iH(1)));
    end

    N_i = zeros(3,size(stheta_iR,1));
    for i = 1:size(stheta_iR,1)
        N_i(:,i)=(1/2)*rho*v_iR(:,i).^2*li(i)*d(i)*C_D_R*stheta_iR(i)^2;
    end
    
    
end

== matlab function tailsitter2019b/Forces/Summation ==
  data: FH_i input; Fa output; FV_i input; MH_i input; MV_i input; N_i input; Ma output; Fr output; Mr output; r_B input; rv_B input; pm input
function [Fa, Ma, Fr, Mr] = fcn(FH_i, FV_i, MH_i, MV_i, N_i, r_B, rv_B, pm)

    Fa = zeros(3,1);
    
    for i = 1:size(FH_i,2)
        Fa = Fa + FH_i(:,i);
    end
    
    for i = 1:size(FV_i,2)
        Fa = Fa + FV_i(:,i);
    end
    
    Ma = zeros(3,1);
    
    for i = 1:size(MH_i,2)
        Ma = Ma + (MH_i(:,i) + cross(r_B(:,i),FH_i(:,i)));
    end
    
    for i = 1:size(MV_i,2)
        Ma = Ma + (MV_i(:,i) + cross(rv_B(:,i),FV_i(:,i)));
    end
    
    Fr = zeros(3,1);
    Mr = zeros(3,1);
    
    for i = 1:size(N_i,2)
        Fr = Fr + N_i(:,i);
        Mr = Mr + cross(pm(:,i),N_i(:,i));
    end


end

== matlab function tailsitter2019b/Forces/Aerodynamics ==
  data: Fa input size=3; tau_a output size=6; Ma input size=3; Fr input size=3; Mr input size=3
function tau_a = fcn(Fa, Ma, Fr, Mr)

    tau_a = zeros(6,1);
    tau_a(1:3) = Fa + Fr;
    tau_a(4:6) = Ma + Mr;

end

== matlab function tailsitter2019b/VR formatting/Euler2Mat5 ==
  data: Theta input; R output
function R = fcn(Theta)
R = eul2rotm(Theta', "ZYX"); %YAW - PITCH - ROLL
end

== matlab function tailsitter2019b/Forces/Thrusters/MATLAB Function ==
  data: F input size=4; FT output size=6
function FT = fcn(F)

    FT = zeros(6,1);
    FT(1) = F(1);
    FT(4:6) = F(2:4);
end

== matlab function tailsitter2019b/Forces/Thrusters/Thrust ==
  data: Omega input; wb input; v_in input; Ith input; rho input; l input; F output size=4; rp input
function F = fcn(Omega, wb, v_in, Ith, rho, l,  rp)
    %Omega(1) = Omega_Left, Omega(2) = Omega_Right
    
    F = Thrust_param(Omega, wb, v_in, Ith, l, rho, rp);
end

== matlab function tailsitter2019b/Forces/Thrusters/Thrust_inv ==
  data: v_in input; wb input; Fp input; rp input; rho input; Ith input; l input; Omega output size=2; Initial_coeffs input
function Omega = fcn(v_in, wb, Fp, rp, rho, Ith, l, Initial_coeffs)
    Omega_init = polyval(Initial_coeffs, Fp(1));
    Omega_init = max(Omega_init, 50);
    Omega_init = [Omega_init; Omega_init];
    Omega_init
    coder. extrinsic('Thrust_inv');
    Omega = zeros(2,1);
    Omega = Thrust_inv(v_in, wb, Fp, rp, rho, Ith, l, Omega_init);
end

== matlab function tailsitter2019b/VR formatting/MATLAB Function ==
  data: NED input; y output; R_eb input
function y = fcn(NED, R_eb)
    R = axang2rotm(R_eb');
    y = inv(R)*NED;
end

== matlab function tailsitter2019b/VR formatting/R*R_in ==
  data: R input; ax_new output; R_in input
function ax_new = fcn(R, R_in)
    ax_new = rotm2axang(R*R_in)';
end

== matlab function tailsitter2019b/VR formatting/R1*R_in ==
  data: R input; ax_new output; R_in input
function ax_new = fcn(R, R_in)
    ax_new = rotm2axang(R*R_in)';
end

== matlab function tailsitter2019b/VR formatting/R_in*R2 ==
  data: R input; ax_new output; R_in input
function ax_new = fcn(R, R_in)
    ax_new = rotm2axang(R_in*R)';
end

== matlab function tailsitter2019b/Forces/Thrusters/Norm of vector ==
  data: v input; v_norm output
function v_norm = fcn(v)
    v_norm = norm(v);
end

== matlab function tailsitter2019b/VR formatting/R_in*R3 ==
  data: R input; ax_new output; R_in input
function ax_new = fcn(R, R_in)
    ax_new = rotm2axang(R_in*R)';
end

== matlab function tailsitter2019b/VR formatting/R_in*R4 ==
  data: R input; ax_new output; R_in input
function ax_new = fcn(R, R_in)
    ax_new = rotm2axang(R_in*R)';
end
